simulink model "control_project_phase1"  (R2015b)
settings: Solver=FixedStepAuto  StartTime=0.0  StopTime=10000  FixedStep=1  RelTol=1e-3
libraries: nesl_utility x6, sh_lib x5, fl_lib x4
settings Model: Creator=asuS  LastModifiedBy=asuS

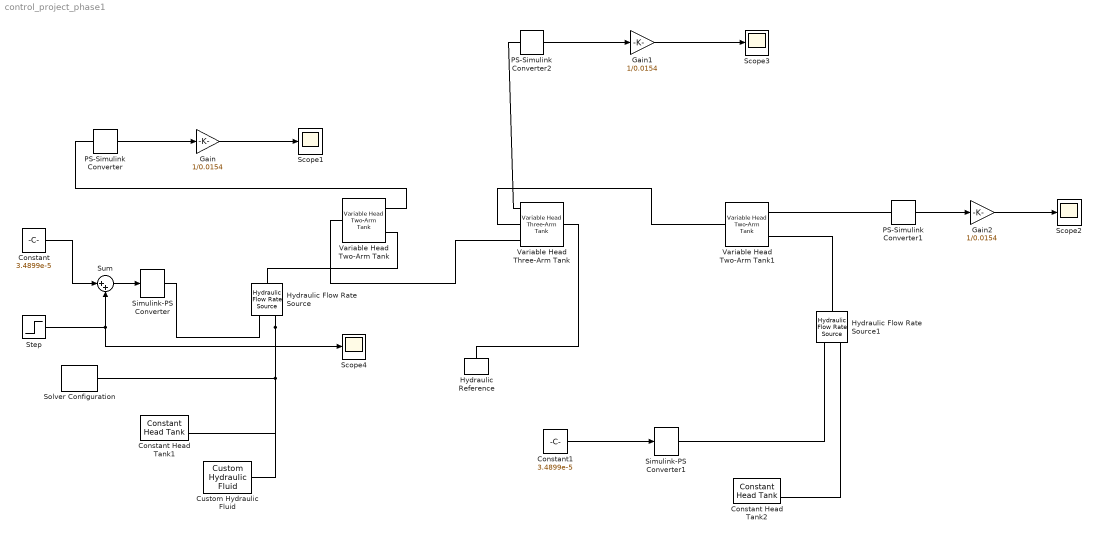
== system control_project_phase1 ==
  Constant : Constant  Value=3.4899e-5
  Constant Head Tank1 : sh_lib/Low-Pressure Blocks/Constant Head Tank  press=0 Pa  fluid_level=100 m  init_volume=0.2 m^3  pipe_diam=0.02 m  loss_coeff=1  gravity_accel=9.80665 m/s^2  pipe_area=0 m^2  C_d=0  p_cr=1 Pa
  Constant Head Tank2 : sh_lib/Low-Pressure Blocks/Constant Head Tank  press=0 Pa  fluid_level=100 m  init_volume=0.2 m^3  pipe_diam=0.02 m  loss_coeff=1  gravity_accel=9.80665 m/s^2  pipe_area=0 m^2  C_d=0  p_cr=1 Pa
  Constant1 : Constant  Value=3.4899e-5
  Custom Hydraulic Fluid : fl_lib/Hydraulic/Hydraulic Utilities/Custom Hydraulic Fluid  density=850 kg/m^3  viscosity_kin=18e-6 m^2/s  bulk=0.8e9 Pa  alpha=0.005  range_error=2
  Gain : Gain  Gain=1/0.0154
  Gain1 : Gain  Gain=1/0.0154
  Gain2 : Gain  Gain=1/0.0154
  Hydraulic Flow Rate Source : fl_lib/Hydraulic/Hydraulic Sources/Hydraulic Flow Rate Source
  Hydraulic Flow Rate Source1 : fl_lib/Hydraulic/Hydraulic Sources/Hydraulic Flow Rate Source
  Hydraulic Reference : fl_lib/Hydraulic/Hydraulic Elements/Hydraulic Reference
  PS-Simulink Converter : nesl_utility/PS-Simulink Converter  PhysicalDomain=network_engine_domain  SubClassName=ps_output  LeftPortType=input  RightPortType=output  PseudoPeriodic=off  Frequencies=[]  Unit=1  AffineConversion=off
  PS-Simulink Converter1 : nesl_utility/PS-Simulink Converter  PhysicalDomain=network_engine_domain  SubClassName=ps_output  LeftPortType=input  RightPortType=output  PseudoPeriodic=off  Frequencies=[]  Unit=1  AffineConversion=off
  PS-Simulink Converter2 : nesl_utility/PS-Simulink Converter  PhysicalDomain=network_engine_domain  SubClassName=ps_output  LeftPortType=input  RightPortType=output  PseudoPeriodic=off  Frequencies=[]  Unit=1  AffineConversion=off
  Scope{1..4} (4 alike) : Scope
  Simulink-PS Converter : nesl_utility/Simulink-PS Converter  PhysicalDomain=network_engine_domain  SubClassName=ps_input  LeftPortType=input  RightPortType=output  PseudoPeriodic=off  Frequencies=[]  NoiseDistribution=none  NoiseParameters=[]  Unit=1  AffineConversion=off  InputFiltering=off  SimscapeFilterOrder=1  InputFilterTimeConstant=0.001  UdotUserProvided=1
  Simulink-PS Converter1 : nesl_utility/Simulink-PS Converter  PhysicalDomain=network_engine_domain  SubClassName=ps_input  LeftPortType=input  RightPortType=output  PseudoPeriodic=off  Frequencies=[]  NoiseDistribution=none  NoiseParameters=[]  Unit=1  AffineConversion=off  InputFiltering=off  SimscapeFilterOrder=1  InputFilterTimeConstant=0.001  UdotUserProvided=1
  Solver Configuration : nesl_utility/Solver Configuration  PhysicalDomain=network_engine_domain  SubClassName=solver  LeftPortType=input  RightPortType=generic  Accelerate=off  Tones=[]  Harmonics=[]  SimulateNoise=off  Profile=off  UseLocalSampling=off  EnableSwitchedLinearOptims=on  FrequencyDomain=off  UseCCode=off  RelTol=0.001  AbsTol=1e-06  MinStep=1e-09  ToWorkspace=off  RevertToSquareIcSolve=off  NumHomotopyIterations=100  PhasorMode=off  PhasorModeNumHarmonics=1  DoDC=off  ResidualTolerance=1e-09  UseLocalSolver=off  LocalSolverChoice=NE_BACKWARD_EULER_ADVANCER  LocalSolverSampleTime=0.001  DoFixedCost=off  MaxNonlinIter=3  MaxModeIter=2  LinearAlgebra=Sparse  DelaysMemoryBudget=1024  AutomaticFiltering=on  FilteringTimeConstant=0.001
  Step : Step  Time=4000  After=0.00001  SampleTime=0
  Sum : Sum  Inputs=|++
  Variable Head Three-Arm Tank : sh_lib/Low-Pressure Blocks/Variable Head Three-Arm Tank  init_volume=0 l  press=0 Pa  level_spec=1  tank_area=0.0154 m^2  fluid_volume_tab=[ 0 0.0028 0.0065 0.0114 0.0176 0.0252 0.0344 0.0436 0.0512 0.0574 0.0623 0.066 0.0688 0.0707 0.07199999999999999 0.0727 ] m^3  fluid_level_tab=[ 0 0.02 0.04 0.06 0.08 0.1 0.12 0.14 0.16 0.18 0.2 0.22 0.24 0.26 0.28 0.3 ] m  pipe_diam_A=5.642e-3 m  loss_coeff_A=1  pipe_diam_B=5.642e-3 m  height_B=0 m  loss_coeff_B=1  pipe_diam_C=6.676e-3 m  height_C=0 m  loss_coeff_C=1  interp_method=1  extrap_method=1
  Variable Head Two-Arm Tank : sh_lib/Low-Pressure Blocks/Variable Head Two-Arm Tank  init_volume=0 l  press=0 Pa  level_spec=1  tank_area=0.0154 m^2  fluid_volume_tab=[ 0 0.0028 0.0065 0.0114 0.0176 0.0252 0.0344 0.0436 0.0512 0.0574 0.0623 0.066 0.0688 0.0707 0.07199999999999999 0.0727 ] m^3  fluid_level_tab=[ 0 0.02 0.04 0.06 0.08 0.1 0.12 0.14 0.16 0.18 0.2 0.22 0.24 0.26 0.28 0.3 ] m  pipe_diam_A=5.642e-3 m  loss_coeff_A=1  pipe_diam_B=5.642e-3 m  height_B=0 m  loss_coeff_B=1  interp_method=1  extrap_method=1
  Variable Head Two-Arm Tank1 : sh_lib/Low-Pressure Blocks/Variable Head Two-Arm Tank  init_volume=0 l  press=0 Pa  level_spec=1  tank_area=0.0154 m^2  fluid_volume_tab=[ 0 0.0028 0.0065 0.0114 0.0176 0.0252 0.0344 0.0436 0.0512 0.0574 0.0623 0.066 0.0688 0.0707 0.07199999999999999 0.0727 ] m^3  fluid_level_tab=[ 0 0.02 0.04 0.06 0.08 0.1 0.12 0.14 0.16 0.18 0.2 0.22 0.24 0.26 0.28 0.3 ] m  pipe_diam_A=5.642e-3 m  loss_coeff_A=1  pipe_diam_B=5.642e-3 m  height_B=0 m  loss_coeff_B=1  interp_method=1  extrap_method=1
  wires:
  PS-Simulink Converter/1 -> Gain/1
  Gain/1 -> Scope1/1
  PS-Simulink Converter2/1 -> Gain1/1
  Gain1/1 -> Scope3/1
  PS-Simulink Converter1/1 -> Gain2/1
  Gain2/1 -> Scope2/1
  Constant1/1 -> Simulink-PS Converter1/1
  Sum/1 -> Simulink-PS Converter/1
  Constant/1 -> Sum/1
  Step/1 -> Sum/2, Scope4/1
  connections:
  Hydraulic Flow Rate Source/RConn2 -- Solver Configuration/RConn1 -- Constant Head Tank1/RConn2 -- Custom Hydraulic Fluid/RConn1
  Variable Head Three-Arm Tank/LConn2 -- Variable Head Two-Arm Tank1/LConn1
  PS-Simulink Converter1/LConn1 -- Variable Head Two-Arm Tank1/RConn1
  Variable Head Three-Arm Tank/RConn1 -- Hydraulic Reference/LConn1
  Hydraulic Flow Rate Source1/LConn1 -- Variable Head Two-Arm Tank1/RConn2
  PS-Simulink Converter2/LConn1 -- Variable Head Three-Arm Tank/LConn1
  Constant Head Tank2/RConn2 -- Hydraulic Flow Rate Source1/RConn2
  Hydraulic Flow Rate Source/LConn1 -- Variable Head Two-Arm Tank/RConn2
  Variable Head Two-Arm Tank/RConn1 -- PS-Simulink Converter/LConn1
  Simulink-PS Converter1/RConn1 -- Hydraulic Flow Rate Source1/RConn1
  Variable Head Two-Arm Tank/LConn1 -- Variable Head Three-Arm Tank/LConn3
  Simulink-PS Converter/RConn1 -- Hydraulic Flow Rate Source/RConn1
